simulink model "signalgeneration"  (Simulink 7.5)
settings: Solver=ode1  StartTime=0.0  StopTime=500  FixedStep=0.1  RelTol=1e-3
libraries: simulink x2
settings Model: Creator=s13071832  LastModifiedBy=s13071832

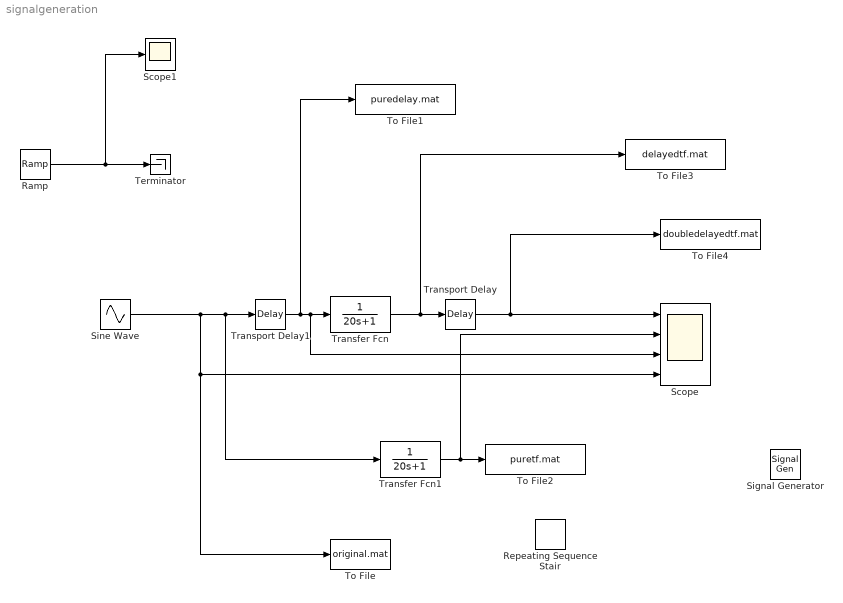
== system signalgeneration ==
  Ramp : simulink/Sources/Ramp  SystemSampleTime=-1  slope=1  start=10  X0=1  VectorParams1D=off
  Repeating Sequence Stair : simulink/Sources/Repeating Sequence Stair  SystemSampleTime=-1  OutValues=[3 1 4 2 1].'  tsamp=-1  OutMin=[]  OutMax=[]  OutDataTypeStr=double  OutputDataTypeScalingMode=double  OutDataType=fixdt(0,8)  ConRadixGroup=Best Precision: Vector-wise  OutScaling=2^-12
  Scope : Scope  NumInputPorts=4
      settings: TimeRange=1000  YMin=-5~-5~-5~-5  YMax=5~5~5~5  MaxDataPoints=10000
  Scope1 : Scope
  Signal Generator : SignalGenerator
  Sine Wave : Sin  Amplitude=1  Bias=0  Frequency=0.5  Phase=0  Samples=10  SampleTime=0  Offset=0
  Terminator : Terminator
  To File : ToFile  Filename=original.mat  MatrixName=original  SaveFormat=Timeseries
  To File1 : ToFile  Filename=puredelay.mat  MatrixName=puredelay  SaveFormat=Timeseries
  To File2 : ToFile  Filename=puretf.mat  MatrixName=puretf  SaveFormat=Timeseries
  To File3 : ToFile  Filename=delayedtf.mat  MatrixName=delayedtf  SaveFormat=Timeseries
  To File4 : ToFile  Filename=doubledelayedtf.mat  MatrixName=doubledelayedtf  SaveFormat=Timeseries
  Transfer Fcn : TransferFcn  Denominator=[20 1]
  Transfer Fcn1 : TransferFcn  Denominator=[20 1]
  Transport Delay : TransportDelay  DelayTime=3
  Transport Delay1 : TransportDelay  DelayTime=6.3
  wires:
  Transfer Fcn/1 -> Transport Delay/1, To File3/1
  Transport Delay/1 -> To File4/1, Scope/1
  Transport Delay1/1 -> To File1/1, Transfer Fcn/1, Scope/3
  Transfer Fcn1/1 -> To File2/1, Scope/2
  Sine Wave/1 -> Transport Delay1/1, Transfer Fcn1/1, To File/1, Scope/4
  Ramp/1 -> Terminator/1, Scope1/1
